simulink model "doc_channel"  (R2014a)
settings: Solver=ode45  SolverMode=SingleTasking  StartTime=0.0  StopTime=inf  RelTol=1e-3
undefined symbols (not defined in the file or in its folder): commblksprivate, Info
libraries: commrandsrc2 x1, commchan3 x1, commsink2 x1
settings Model: Creator=The MathWorks Inc.
settings DataIOCC: SignalLoggingSaveFormat=ModelDataLogs  SaveOutput=off  SaveTime=off  SignalLoggingName=sigsOut
settings OptimizationCC: BooleanDataType=off  InlineParams=on  ExpressionDepthLimit=2147483647
settings DebuggingCC: AlgebraicLoopMsg=error  SaveWithParameterizedLinksMsg=none  UnderspecifiedInitializationDetection=Classic  SignalResolutionControl=TryResolveAllWithWarning  SolverPrmCheckMsg=none  MultiTaskDSMMsg=warning  MultiTaskCondExecSysMsg=none  FcnCallInpInsideContextMsg=UseLocalSettings  StateNameClashWarn=warning  StrictBusMsg=None
settings HardwareCC: TargetUnknown=on
settings RTWCC: IncludeERTFirstTime=on
settings GRTTargetCC: CombineOutputUpdateFcns=off  GRTInterface=on

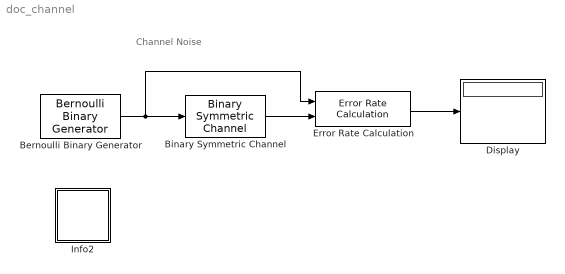
== system doc_channel ==
  note: Channel Noise
  " Display" : Display
  Bernoulli Binary Generator : commrandsrc2/Bernoulli Binary Generator  P=0.5  seed=61  Ts=1  frameBased=off  sampPerFrame=1  orient=off  outDataType=double
  Binary Symmetric Channel : commchan3/Binary Symmetric Channel  P=0.01  s=2137  E=off  outDtype=double
  Error Rate Calculation : commsink2/Error Rate Calculation  N=0  st_delay=0  cp_mode=Entire frame  subframe=[]  PMode=Port  WsName=ErrorVec  RsMode2=off  stop=on  numErr=100  maxBits=1e6
  Info2 : Subsystem  AncestorBlock=commblksprivate/Info  mask(Info){}
      settings: OpenFcn=helpview([docroot '/toolbox/comm/comm.map'], 'doc_channel')
      mask Display: disp('Info')
  wires:
  Error Rate Calculation/1 -> " Display"/1
  Bernoulli Binary Generator/1 -> Error Rate Calculation/1, Binary Symmetric Channel/1
  Binary Symmetric Channel/1 -> Error Rate Calculation/2

== system doc_channel/Info2 ==
